simulink model "energy_tracker"  (R2025b)
settings: Solver=VariableStepAuto  StartTime=0.0  StopTime=10.0  RelTol=1e-3
undefined symbols (not defined in the file or in its folder): DiscIntNeverNeededParam
settings Model: Creator=samue  LastModifiedBy=samue

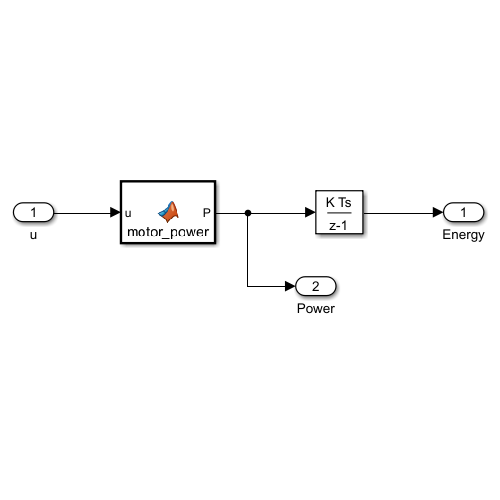
[thumbnail: Simulink's stored preview of the top-level diagram]
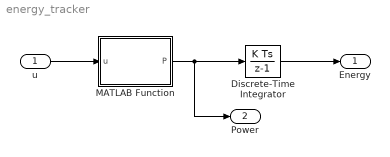
== system energy_tracker ==
  u : Inport
  Discrete-Time Integrator : DiscreteIntegrator  SampleTime=-1  ICPrevOutput=DiscIntNeverNeededParam  ICPrevScaledInput=DiscIntNeverNeededParam
  MATLAB Function : MATLAB Function  TreatAsAtomicUnit=on
  Energy : Outport
  Power : Outport  Port=2
  wires:
  u/1 -> MATLAB Function/1(u)
  MATLAB Function/1(P) -> Discrete-Time Integrator/1, Power/1
  Discrete-Time Integrator/1 -> Energy/1

== matlab function energy_tracker/MATLAB Function ==
  data: u input; P output
function P = motor_power(u)
% Calculates motor power usage based on throttle
    P = 0; % needs table to be implemented
end
